simulink model "arte"  (R2013b)
(part 2 of 27)

  pre_dedisp_delay10/2(dout_valid) -> dedispersor10/3(din_valid)
  pre_dedisp_delay10/1(Out1) -> dedispersor10/2(din)
  [rst_dedisp] -> dedispersor10/1(rst)
  dedispersor10/1(integ_pow) -> post_dedisp_conv10/1(din)
  dedispersor10/2(integ_valid) -> post_dedisp_conv10/2(din_valid)
  post_dedisp_conv10/1(dout) -> post_dedisp_delay10/1(In1)
  post_dedisp_conv10/2(dout_valid) -> post_dedisp_delay10/2(din_valid)
  post_dedisp_delay10/1(Out1) -> Convert39/1, Relational15/1, mov_avg10/2(din)
  [rst_dedisp] -> mov_avg10/1(rst)
  mov_avg10/1(dout) -> add_stat10/2
  add_stat10/1 -> Relational15/2, Convert40/1
  [theta10] -> add_stat10/1
  [rst_detection] -> Register28/2
  Register28/1 -> [detection10]
  Counter31/1 -> dedisp10/1(addr)
  post_dedisp_delay10/2(dout_valid) -> mov_avg10/3(din_valid), Counter31/1, pipeline95/1(d), dedisp10/3(we)
  Convert39/1 -> Reinterpret54/1
  Reinterpret54/1 -> dedisp10/2(data_in)
  Counter32/1 -> avg10/1(addr)
  mov_avg10/2(dout_valid) -> Counter32/1, avg10/3(we)
  Convert40/1 -> Reinterpret55/1
  Reinterpret55/1 -> avg10/2(data_in)
  pipeline74/1 -> Register28/3, Register28/1
  Logical43/1 -> pipeline74/1
  Relational15/1 -> Logical43/2
  [rfi_detected] -> Inverter13/1
  Logical44/1 -> Register27/3, Register27/1, enabled_vacc10/1(new_acc)
  acc_cntrl15/1(new_acc) -> Logical44/2
  [en_dedisp] -> Logical44/1
  Register27/1 -> Logical45/1
  [rst_dedisp] -> Register27/2
  Logical45/1 -> enabled_vacc10/3(din_valid)
  pipeline72/1(q) -> Logical45/2
  [detection10] -> Logical3/11
  control/31(acc_len11) -> [acc_len10]
  control/45(theta11) -> [theta10]
  control/46(theta12) -> [theta11]
  control/32(acc_len12) -> [acc_len11]
  [detection9] -> Concat9/2
  [detection8] -> Concat9/3
  [detection7] -> Concat9/4
  [detection6] -> Concat9/5
  [detection5] -> Concat9/6
  [detection4] -> Concat9/7
  [detection3] -> Concat9/8
  [detection2] -> Concat9/9
  [detection1] -> Concat9/10
  [detection0] -> Concat9/11
  [detection10] -> Concat9/1
  Inverter2/1 -> Logical11/3
  pipeline75/1(q) -> Logical11/1
  Inverter4/1 -> Logical12/3
  pipeline79/1(q) -> Logical12/1
  Inverter5/1 -> Logical13/3
  pipeline80/1(q) -> Logical13/1
  Inverter6/1 -> Logical14/3
  pipeline83/1(q) -> Logical14/1
  Inverter7/1 -> Logical15/3
  pipeline84/1(q) -> Logical15/1
  Inverter8/1 -> Logical28/3
  pipeline87/1(q) -> Logical28/1
  Inverter9/1 -> Logical31/3
  pipeline88/1(q) -> Logical31/1
  Inverter10/1 -> Logical34/3
  pipeline90/1(q) -> Logical34/1
  Inverter11/1 -> Logical37/3
  pipeline92/1(q) -> Logical37/1
  Inverter12/1 -> Logical40/3
  pipeline93/1(q) -> Logical40/1
  Inverter13/1 -> Logical43/3
  pipeline95/1(q) -> Logical43/1
  control/51(noise_diode) -> [noise_diode]
  [noise_diode] -> pipeline96/1
  pipeline96/1 -> noise_diode/1
  [ovf_rst] -> adc_clip0/1(rst)
  adc_clip0/1(clip) -> pipeline99/1(d)
  Relational16/1 -> pipeline105/1(d), Counter/1
  Counter/1 -> Relational16/1
  [acc_len] -> Shift/1
  Reinterpret/1 -> [ovf_rst]
  Convert41/1 -> Concat5/4
  [detection0] -> Concat10/1
  [detection1] -> Concat10/2
  [detection2] -> Concat10/3
  [detection3] -> Concat10/4
  [detection4] -> Concat10/5
  [detection5] -> Concat10/6
  [detection6] -> Concat10/7
  [detection7] -> Concat10/8
  [detection8] -> Concat10/9
  [detection9] -> Concat10/10
  [detection10] -> Concat10/11
  [clip3] -> Concat10/12
  [clip2] -> Concat10/13
  [clip1] -> Concat10/14
  [clip0] -> Concat10/15
  pipeline99/1(q) -> [clip0]
  pipeline105/1(q) -> Reinterpret/1
  Shift/1 -> Relational16/2
  pipeline106/1(q) -> Convert41/1
  timestamp/1(in_reg) -> AddSub/2, Relational18/2
  Counter33/1 -> Relational17/1
  Relational17/1 -> Counter33/1, Counter34/2
  Constant5/1 -> Relational17/2
  Constant7/1 -> Relational18/1
  Relational18/1 -> Counter34/1
  Counter34/1 -> AddSub/1
  [fft0_0] -> beam_post_complex_add/2(In1)
  [sync_out0] -> beam_post_complex_add/1(sync_in)
  [fft0_1] -> beam_post_complex_add/3(In2)
  [fft0_2] -> beam_post_complex_add/4(In3)
  [fft0_3] -> beam_post_complex_add/5(In4)
  Constant2/1 -> [adc2], [adc1]
  Constant3/1 -> [clip3], [clip2], [clip1]
  Constant9/1 -> [rfi_detected]
